simulink model "Lab2"  (Simulink 8.8)
settings: Solver=FixedStepAuto  StartTime=0.0  StopTime=0.5  FixedStep=0.001  MaxStep=10^(-3)  RelTol=1e-3  EnableMultiTasking=on
settings Model: Creator=student  LastModifiedBy=Admin
settings OptimizationCC: ExpressionDepthLimit=2147483647  InitFltsAndDblsToZero=on
settings DebuggingCC: SaveWithParameterizedLinksMsg=none  SolverPrmCheckMsg=warning
settings GRTTargetCC: TargetFcnLib=ansi_tfl_tmw.mat  GeneratePreprocessorConditionals=Use local settings

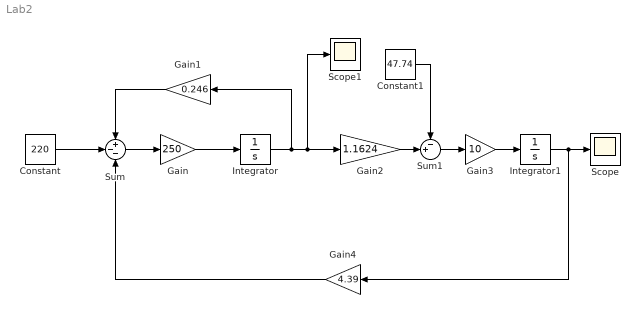
== system Lab2 ==
  Constant : Constant  Value=220
  Constant1 : Constant  Value=47.74
  Gain : Gain  Gain=250
  Gain1 : Gain  Gain=0.246
  Gain2 : Gain  Gain=1.1624
  Gain3 : Gain  Gain=10
  Gain4 : Gain  Gain=4.39
  Integrator : Integrator
  Integrator1 : Integrator
  Scope : Scope
  Scope1 : Scope
  Sum : Sum  Inputs=+--
  Sum1 : Sum  Inputs=-+|
  wires:
  Gain3/1 -> Integrator1/1
  Constant/1 -> Sum/2
  Sum/1 -> Gain/1
  Gain/1 -> Integrator/1
  Integrator/1 -> Gain1/1, Scope1/1, Gain2/1
  Gain2/1 -> Sum1/2
  Sum1/1 -> Gain3/1
  Integrator1/1 -> Gain4/1, Scope/1
  Gain4/1 -> Sum/3
  Gain1/1 -> Sum/1
  Constant1/1 -> Sum1/1
